simulink model "simscape_final"  (R2023a)
settings: Solver=ode23tb  StartTime=0.0  StopTime=0.15  RelTol=1e-3
PreLoadFcn:
  | clear;
  | clc;
  | %load('70PVArrayExperimentalData.mat');
  | 
  | MPPT_IncCond=Simulink.Variant('MPPT_MODE==1')
  | MPPT_PandO=Simulink.Variant('MPPT_MODE==2')
  | 
  | MPPT_MODE=2
  | 
  | 
  | Constant_800=Simulink.Variant('Irradiance_Mode==1')
  | Constant_1000=Simulink.Variant('Irradiance_Mode==2')
  | Step=Simulink.Variant('Irradiance_Mode==3')
  | Step2=Simulink.Variant('Irradiance_Mode==4')
  | Irradiance_Mode=4
values from neighbouring files (symbols this model uses):
  ArrayCurrent2 = [3.444 3.44193327944 3.44169340802 3.44145256796 3.44121172825 3.44097088836 3.44073004827 3.44048920799 3.4402483675 3.44000752679 3.43976668584 3.43952584466 ... (5005 elements, 385x13)]    [InitPVArrayData.mat]
  ArrayVoltage = [0 0.1 0.2 0.3 0.4 0.5 0.6 0.7 0.8 0.9 1 1.1 ... (215 elements, 1x215)]    [25PVArrayExperimentalData.mat]    (also in 70PVArrayExperimentalData.mat = [0 0.1 0.2 0.3 0.4 0.5 0.6 0.7 0.8 0.9 1 1.1 ... (183 elemen; InitPVArrayData.mat = [0 0.1 0.2 0.3 0.4 0.5 0.6 0.7 0.8 0.9 1 1.1 ... (385 elemen)
  Irradiance = [400 450 500 550 600 650 700 750 800 850 900 950 ... (17 elements, 1x17)]    [25PVArrayExperimentalData.mat]    (also in 70PVArrayExperimentalData.mat; InitPVArrayData.mat = [400 450 500 550 600 650 700 750 800 850 900 950 ... (13 ele)
undefined symbols (not defined in the file or in its folder): sigbuilder_block
libraries: spsSeriesRLCBranchLib x6, SignalEditorBlockLib x4, spsVoltageMeasurementLib x4, simulink x3, spsDiodeLib x3, spsMosfetLib x3, spsCurrentMeasurementLib x2, spsControlledCurrentSourceLib x2, spspowerguiLib x1
settings Model: SimulationMode=accelerator  Creator=gabrielcrisan  LastModifiedBy=gabrielcrisan

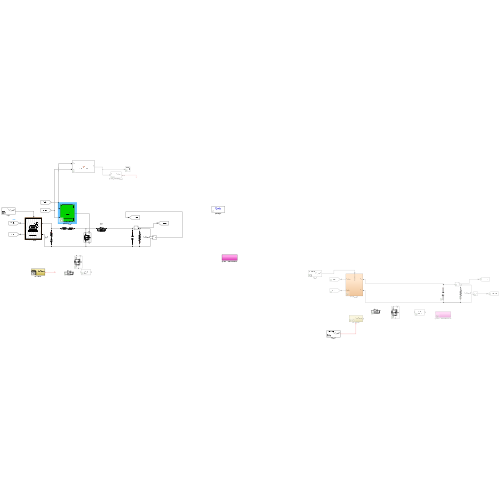
[thumbnail: Simulink's stored preview of the top-level diagram]
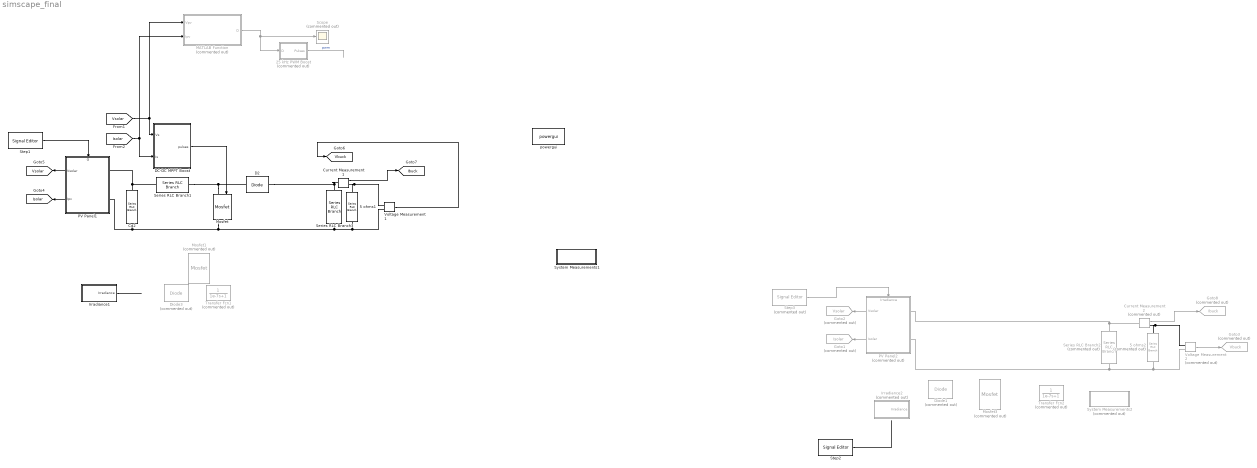
== system simscape_final ==
  25 kHz PWM Boost : Subsystem  Commented=on  mask{Freq=25000}
      mask prompts: Freq "Frequency (Hz)"
  5 ohms1 : spsSeriesRLCBranchLib/Series RLC Branch  LConnTagsString=__new0  RConnTagsString=__new0  BranchType=R  Resistance=15  Inductance=0  SetiL0=off  InitialCurrent=0  Capacitance=100e-6  Setx0=off  InitialVoltage=0  Measurements=Branch voltage and current
  5 ohms2 : spsSeriesRLCBranchLib/Series RLC Branch  Commented=on  LConnTagsString=__new0  RConnTagsString=__new0  BranchType=R  Resistance=15  Inductance=0  SetiL0=off  InitialCurrent=0  Capacitance=100e-6  Setx0=off  InitialVoltage=0  Measurements=Branch voltage and current
  Cg2 : spsSeriesRLCBranchLib/Series RLC Branch  LConnTagsString=__new0  RConnTagsString=__new0  BranchType=RC  Resistance=0.000001  Inductance=0  SetiL0=off  InitialCurrent=0  Capacitance=100e-6  Setx0=off  InitialVoltage=0  Measurements=None
  Current Measurement1 : spsCurrentMeasurementLib/Current Measurement  PhasorSimulation=off  OutputType=Complex  PSBequivalent=0
  Current Measurement2 : spsCurrentMeasurementLib/Current Measurement  Commented=on  PhasorSimulation=off  OutputType=Complex  PSBequivalent=0
  D2 : spsDiodeLib/Diode  Ron=0.001  Lon=0  Vf=0.8  IC=0  UseSnubber=off  Rs=500  Cs=250e-9  Measurements=off
  DC-DC MPPT Boost : Subsystem  Variant=on
      mask Display: image('$imagefile'); % Use "Edit Image" on toolstrip to change.
  Diode1 : spsDiodeLib/Diode  Commented=on  Ron=0.001  Lon=0  Vf=0.8  IC=0  UseSnubber=0  Rs=500  Cs=250e-9  Measurements=off
  Diode3 : spsDiodeLib/Diode  Commented=on  Ron=0.001  Lon=0  Vf=0.8  IC=0  UseSnubber=0  Rs=500  Cs=250e-9  Measurements=off
  Goto1 : Goto  Commented=on  GotoTag=Isolar  TagVisibility=global
  Goto2 : Goto  Commented=on  GotoTag=Vsolar  TagVisibility=global
  Goto3 : Goto  Commented=on  GotoTag=Vbuck  TagVisibility=global
  Goto8 : Goto  Commented=on  GotoTag=Ibuck  TagVisibility=global
  Irradiance1 : Subsystem  Variant=on
  Irradiance2 : Subsystem  Commented=on  Variant=on
  MATLAB Function : MATLAB Function  Commented=on  TreatAsAtomicUnit=on
  Mosfet : spsMosfetLib/Mosfet  Ron=0.001  Lon=0  Rd=0.001  Vfd=0  IC=0  Rs=1e5  Cs=inf  Measurements=on
  Mosfet1 : spsMosfetLib/Mosfet  Commented=on  Ron=0.1  Lon=0  Rd=0.01  Vfd=0  IC=0  Rs=1e5  Cs=inf  Measurements=off
  Mosfet3 : spsMosfetLib/Mosfet  Commented=on  Ron=0.1  Lon=0  Rd=0.01  Vfd=0  IC=0  Rs=1e5  Cs=inf  Measurements=off
  PV Panel1 : Subsystem
      settings: PortSchema="{\"entries\":[{\"content\":{\"sides\":[{\"content\":{\"connectorIds\":[\"LConn1\",\"LConn2\"]},\"type\":\"ConnectorPlacement.EquallySpacedRectSide\",\"uuid\":\"43992eb9-8484-404f-bfb9-e76ffbcbe789\"},{\"content\":{\"connectorIds\":[\"Out1\",\"Out2\"],\"side\":\"RIGHT\"},\"type\":\"ConnectorPlacement.EquallySpacedRectSide\",\"uuid\":\"a1e110c3-733a-48a0-9f21-72c7769fefeb\"},{\"content\":{\"connectorIds\":[\"In1\"],\"side\":\"TOP\"},\"type\":\"ConnectorPlacement.EquallySpacedRectSide\",\"uuid\":\"462cd67a-8eaa-46f4-b7ed-de8fc592bb6c\"}]},\"type\":\"ConnectorPlacement.EquallySpacedConnector\",\"uuid\":\"36390758-a197-45c1-a178-dbe841a9808e\"}],\"packageUris\":[\"http://schema.mathworks.com/mf0/Connector/R2020b\"],\"version\":\"1.0\"}"
      mask Display: image('$imagefile'); % Use "Edit Image" on toolstrip to change.
  PV Panel2 : Subsystem  Commented=on
      settings: PortSchema="{\"entries\":[{\"content\":{\"sides\":[{\"content\":{\"connectorIds\":[\"LConn1\",\"LConn2\"]},\"type\":\"ConnectorPlacement.EquallySpacedRectSide\",\"uuid\":\"d9bf1892-3ed2-4c2d-93df-cd3e3a16e4c3\"},{\"content\":{\"connectorIds\":[\"Out1\",\"Out2\"],\"side\":\"RIGHT\"},\"type\":\"ConnectorPlacement.EquallySpacedRectSide\",\"uuid\":\"0c4558bb-5c04-452d-a739-3e65dffd873d\"},{\"content\":{\"connectorIds\":[\"In1\"],\"side\":\"TOP\"},\"type\":\"ConnectorPlacement.EquallySpacedRectSide\",\"uuid\":\"688d7f81-1212-47ef-a811-baa40651be20\"}]},\"type\":\"ConnectorPlacement.EquallySpacedConnector\",\"uuid\":\"9406dafc-96f7-4a37-8af1-81987149706d\"}],\"packageUris\":[\"http://schema.mathworks.com/mf0/Connector/R2020b\"],\"version\":\"1.0\"}"
  Scope : Scope  Commented=on
  Series RLC Branch1 : spsSeriesRLCBranchLib/Series RLC Branch  LConnTagsString=__new0  RConnTagsString=__new0  BranchType=RL  Resistance=0.001  Inductance=200e-6  SetiL0=off  InitialCurrent=0  Capacitance=100e-6  Setx0=off  InitialVoltage=0  Measurements=None
  Series RLC Branch2 : spsSeriesRLCBranchLib/Series RLC Branch  Commented=on  LConnTagsString=__new0  RConnTagsString=__new0  BranchType=C  Resistance=1e-6  Inductance=0  SetiL0=off  InitialCurrent=0  Capacitance=50e-6  Setx0=off  InitialVoltage=0  Measurements=None
  Series RLC Branch3 : spsSeriesRLCBranchLib/Series RLC Branch  LConnTagsString=__new0  RConnTagsString=__new0  BranchType=C  Resistance=1e-6  Inductance=0  SetiL0=off  InitialCurrent=0  Capacitance=50e-6  Setx0=off  InitialVoltage=0  Measurements=None
  Step1 : SignalEditorBlockLib/Signal Editor  VariantControl=Choice  FileName=IR_scenario.mat  ActiveScenario=Scenario  ActiveSignal=Ir1_rand  IsBus=off  OutputBusObjectStr=Bus: BusObject  SampleTime=0  Interpolate=off  ZeroCross=off  OutputAfterFinalValue=Setting to zero  Unit=inherit  PreserveSignalName=on  ApplySigPropsToAllScenarios=on
  Step2 : SignalEditorBlockLib/Signal Editor  VariantControl=Choice  FileName=IR_scenario.mat  ActiveScenario=Scenario  ActiveSignal=Ir1_rand  IsBus=off  OutputBusObjectStr=Bus: BusObject  SampleTime=0  Interpolate=off  ZeroCross=off  OutputAfterFinalValue=Setting to zero  Unit=inherit  PreserveSignalName=on  ApplySigPropsToAllScenarios=on
  Step3 : SignalEditorBlockLib/Signal Editor  Commented=on  VariantControl=Choice  FileName=IR_scenario.mat  ActiveScenario=Scenario  ActiveSignal=Ir1_rand  IsBus=off  OutputBusObjectStr=Bus: BusObject  SampleTime=0  Interpolate=off  ZeroCross=off  OutputAfterFinalValue=Setting to zero  Unit=inherit  PreserveSignalName=on  ApplySigPropsToAllScenarios=on
  System Measurements1 : Subsystem
  System Measurements2 : Subsystem  Commented=on
  Transfer Fcn1 : TransferFcn  Commented=on  Denominator=[1e-7 1]
  Transfer Fcn2 : TransferFcn  Commented=on  Denominator=[1e-7 1]
  Voltage Measurement1 : spsVoltageMeasurementLib/Voltage Measurement  PhasorSimulation=off  OutputType=Complex  PSBequivalent=0
  Voltage Measurement2 : spsVoltageMeasurementLib/Voltage Measurement  Commented=on  PhasorSimulation=off  OutputType=Complex  PSBequivalent=0
  powergui : spspowerguiLib/powergui  Priority=1  SimulationMode=Discrete  SampleTime=1e-7  frequency=60  Iterations=50  frequencyindice=0  Pbase=100e6  ErrMax=1e-4  UnitsV=kV  UnitsW=MW  buscounter=0  FunctionMessages=off  echomessages=off  EnableUseOfTLC=off  CurrentSourceSwitches=off  DisableSnubberDevices=off  DisableRonSwitches=off  DisableVfSwitches=off  DisplayEquations=off  AutomaticDiscreteSolvers=off  SolverType=Tustin/Backward Euler (TBE)  Interpol=off  ExternalGateDelay=off  methode=off  Ts=100  x0status=blocks  SPID=on  SwTol=0  HookPort=off  NonlinearTolerance=1e-4  nMaxIteration=100  ContinueOnMaxIteration=off  RestoreLinks=warning  ResistiveCurrentMeasurement=off  Frange=[0:2:500]  Ylog=off  Xlog=on  ShowGrid=off  save=off  variable=ZData  structure=0  ZoomFFT=off  StartTime=0.0  cycles=1  DisplayStyle=1  fundamental=60  FreqAxis=off  MaxFrequency=1000  frequencyindicesteady=1  RmsSteady=1  display=off
  tag scope: Ibuck=global, Isolar=global, Vbuck=global, Vsolar=global
  wires:
  [Vsolar] -> MATLAB Function/1(Vpv), DC-DC MPPT Boost/1(Vs)
  PV Panel1/1(Vsolar) -> [Vsolar]
  Irradiance1/1(Irradiance) -> ?
  MATLAB Function/1(D) -> Scope/1, 25 kHz PWM Boost/1(D)
  [Isolar] -> MATLAB Function/2(Ipv), DC-DC MPPT Boost/2(Is)
  Voltage Measurement1/1 -> [Vbuck]
  Current Measurement1/1 -> [Ibuck]
  PV Panel1/2(Ipv) -> [Isolar]
  25 kHz PWM Boost/1(Pulses) -> ?  "pwm"
  DC-DC MPPT Boost/1(pulses) -> Mosfet/1
  PV Panel2/1(Vsolar) -> Goto2/1
  PV Panel2/2(Isolar) -> Goto1/1
  Voltage Measurement2/1 -> Goto3/1
  Current Measurement2/1 -> Goto8/1
  Step2/1 -> ?
  Step1/1 -> PV Panel1/1(G)
  Step3/1 -> PV Panel2/1(Irradiance)
  connections:
  PV Panel1/LConn2 -- Cg2/RConn1 -- Mosfet/RConn1 -- 5 ohms1/LConn1 -- Voltage Measurement1/LConn2 -- Series RLC Branch3/RConn1
  PV Panel1/LConn1 -- Series RLC Branch1/RConn1 -- Cg2/LConn1
  D2/RConn1 -- Series RLC Branch3/LConn1 -- Current Measurement1/LConn1
  Mosfet/LConn1 -- Series RLC Branch1/LConn1 -- D2/LConn1
  Voltage Measurement1/LConn1 -- 5 ohms1/RConn1 -- Current Measurement1/RConn1
  Current Measurement2/LConn1 -- PV Panel2/LConn1 -- Series RLC Branch2/LConn1
  Voltage Measurement2/LConn1 -- 5 ohms2/RConn1 -- Current Measurement2/RConn1
  Voltage Measurement2/LConn2 -- 5 ohms2/LConn1 -- Series RLC Branch2/RConn1 -- PV Panel2/LConn2

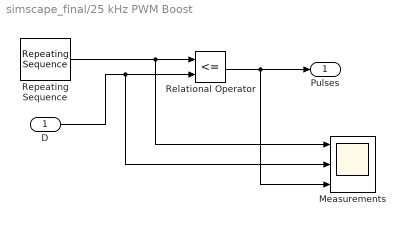
== system simscape_final/25 kHz PWM Boost ==
  D : Inport
  Measurements : Scope  NumInputPorts=3
  Relational Operator : RelationalOperator  Operator=<=  OutDataTypeStr=boolean  ZeroCross=off  InputSameDT=off
  Repeating Sequence : simulink/Sources/Repeating Sequence  rep_seq_t="[0  1/Freq]"  rep_seq_y=[0 1]
  Pulses : Outport
  wires:
  Repeating Sequence/1 -> Measurements/1, Relational Operator/1
  Relational Operator/1 -> Measurements/3, Pulses/1
  D/1 -> Measurements/2, Relational Operator/2

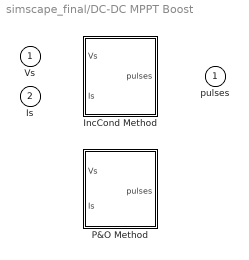
== system simscape_final/DC-DC MPPT Boost ==
  Vs : Inport
  Is : Inport  Port=2
  IncCond Method : Subsystem  VariantControl=MPPT_IncCond
  P&O Method : Subsystem  VariantControl=MPPT_PandO
  pulses : Outport

== system simscape_final/Irradiance1 ==
  Constant 1000 : Subsystem  Tag=STV Subsys  LoadFcn=sigbuilder_block('load');  StartFcn=sigbuilder_block('start');  StopFcn=sigbuilder_block('stop');  ClipboardFcn=sigbuilder_block('clipboard');  VariantControl=Constant_1000  mask(Sigbuilder block){tuvar=[0:10]}
      mask help: Simulink:masks:SigbuilderBlock_MD
      mask init:
      | if ~strcmp(get_param(bdroot(gcbh),'SimulationStatus'),'stopped') tuvar = sigbuilder_block('maskInit'); end
      settings: CopyFcn=sigbuilder_block('copy');  DeleteFcn=sigbuilder_block('delete');  ModelCloseFcn=sigbuilder_block('modelClose');  PreSaveFcn=sigbuilder_block('preSave');  PauseFcn=sigbuilder_block('pause')  ContinueFcn=sigbuilder_block('continue')  NameChangeFcn=sigbuilder_block('namechange');  OpenFcn=sigbuilder_block('open',[365.25 126 411.75 327.75 ]);  CloseFcn=sigbuilder_block('close');
      mask Display: plot(0, 0, 100, 100,[2, 2, 32, 32, 2], [68, 8, 8, 68, 68],[32, 2], [38, 38], [32, 19, 2],[53, 60, 44], [32, 17, 17, 2],[16, 16, 31, 31]);txt = getActiveGroup(gcbh);text(2, 100, txt,'verticalAlignment', 'top');
  "Constant 800 " : Subsystem  Tag=STV Subsys  LoadFcn=sigbuilder_block('load');  StartFcn=sigbuilder_block('start');  StopFcn=sigbuilder_block('stop');  ClipboardFcn=sigbuilder_block('clipboard');  VariantControl=Constant_800  mask(Sigbuilder block){tuvar=[0:10]}
      mask help: Simulink:masks:SigbuilderBlock_MD
      mask init:
      | if ~strcmp(get_param(bdroot(gcbh),'SimulationStatus'),'stopped') tuvar = sigbuilder_block('maskInit'); end
      settings: CopyFcn=sigbuilder_block('copy');  DeleteFcn=sigbuilder_block('delete');  ModelCloseFcn=sigbuilder_block('modelClose');  PreSaveFcn=sigbuilder_block('preSave');  PauseFcn=sigbuilder_block('pause')  ContinueFcn=sigbuilder_block('continue')  NameChangeFcn=sigbuilder_block('namechange');  OpenFcn=sigbuilder_block('open',[365.25 126 411.75 327.75 ]);  CloseFcn=sigbuilder_block('close');
      mask Display: plot(0, 0, 100, 100,[2, 2, 32, 32, 2], [68, 8, 8, 68, 68],[32, 2], [38, 38], [32, 19, 2],[53, 60, 44], [32, 17, 17, 2],[16, 16, 31, 31]);txt = getActiveGroup(gcbh);text(2, 100, txt,'verticalAlignment', 'top');
  Step : Subsystem  Tag=STV Subsys  LoadFcn=sigbuilder_block('load');  StartFcn=sigbuilder_block('start');  StopFcn=sigbuilder_block('stop');  ClipboardFcn=sigbuilder_block('clipboard');  VariantControl=Step  mask(Sigbuilder block){tuvar=[0:10]}
      mask help: Simulink:masks:SigbuilderBlock_MD
      mask init:
      | if ~strcmp(get_param(bdroot(gcbh),'SimulationStatus'),'stopped') tuvar = sigbuilder_block('maskInit'); end
      settings: CopyFcn=sigbuilder_block('copy');  DeleteFcn=sigbuilder_block('delete');  ModelCloseFcn=sigbuilder_block('modelClose');  PreSaveFcn=sigbuilder_block('preSave');  PauseFcn=sigbuilder_block('pause')  ContinueFcn=sigbuilder_block('continue')  NameChangeFcn=sigbuilder_block('namechange');  OpenFcn=sigbuilder_block('open',[135.75 161.25 411.75 327.75 ]);  CloseFcn=sigbuilder_block('close');
      mask Display: plot(0, 0, 100, 100,[2, 2, 32, 32, 2], [68, 8, 8, 68, 68],[32, 2], [38, 38], [32, 19, 2],[53, 60, 44], [32, 17, 17, 2],[16, 16, 31, 31]);txt = getActiveGroup(gcbh);text(2, 100, txt,'verticalAlignment', 'top');
  Irradiance : Outport

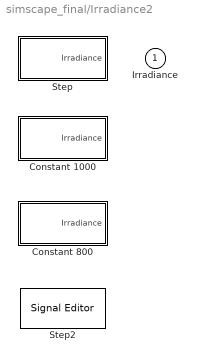
== system simscape_final/Irradiance2 ==
  Constant 1000 : Subsystem  Tag=STV Subsys  LoadFcn=sigbuilder_block('load');  StartFcn=sigbuilder_block('start');  StopFcn=sigbuilder_block('stop');  ClipboardFcn=sigbuilder_block('clipboard');  VariantControl=Constant_1000  mask(Sigbuilder block){tuvar=[0:10]}
      mask help: Simulink:masks:SigbuilderBlock_MD
      mask init:
      | if ~strcmp(get_param(bdroot(gcbh),'SimulationStatus'),'stopped') tuvar = sigbuilder_block('maskInit'); end
      settings: CopyFcn=sigbuilder_block('copy');  DeleteFcn=sigbuilder_block('delete');  ModelCloseFcn=sigbuilder_block('modelClose');  PreSaveFcn=sigbuilder_block('preSave');  PauseFcn=sigbuilder_block('pause')  ContinueFcn=sigbuilder_block('continue')  NameChangeFcn=sigbuilder_block('namechange');  OpenFcn=sigbuilder_block('open',[365.25 126 411.75 327.75 ]);  CloseFcn=sigbuilder_block('close');
      mask Display: plot(0, 0, 100, 100,[2, 2, 32, 32, 2], [68, 8, 8, 68, 68],[32, 2], [38, 38], [32, 19, 2],[53, 60, 44], [32, 17, 17, 2],[16, 16, 31, 31]);txt = getActiveGroup(gcbh);text(2, 100, txt,'verticalAlignment', 'top');
  "Constant 800 " : Subsystem  Tag=STV Subsys  LoadFcn=sigbuilder_block('load');  StartFcn=sigbuilder_block('start');  StopFcn=sigbuilder_block('stop');  ClipboardFcn=sigbuilder_block('clipboard');  VariantControl=Constant_800  mask(Sigbuilder block){tuvar=[0:10]}
      mask help: Simulink:masks:SigbuilderBlock_MD
      mask init:
      | if ~strcmp(get_param(bdroot(gcbh),'SimulationStatus'),'stopped') tuvar = sigbuilder_block('maskInit'); end
      settings: CopyFcn=sigbuilder_block('copy');  DeleteFcn=sigbuilder_block('delete');  ModelCloseFcn=sigbuilder_block('modelClose');  PreSaveFcn=sigbuilder_block('preSave');  PauseFcn=sigbuilder_block('pause')  ContinueFcn=sigbuilder_block('continue')  NameChangeFcn=sigbuilder_block('namechange');  OpenFcn=sigbuilder_block('open',[365.25 126 411.75 327.75 ]);  CloseFcn=sigbuilder_block('close');
      mask Display: plot(0, 0, 100, 100,[2, 2, 32, 32, 2], [68, 8, 8, 68, 68],[32, 2], [38, 38], [32, 19, 2],[53, 60, 44], [32, 17, 17, 2],[16, 16, 31, 31]);txt = getActiveGroup(gcbh);text(2, 100, txt,'verticalAlignment', 'top');
  Step : Subsystem  Tag=STV Subsys  LoadFcn=sigbuilder_block('load');  StartFcn=sigbuilder_block('start');  StopFcn=sigbuilder_block('stop');  ClipboardFcn=sigbuilder_block('clipboard');  VariantControl=Step  mask(Sigbuilder block){tuvar=[0:10]}
      mask help: Simulink:masks:SigbuilderBlock_MD
      mask init:
      | if ~strcmp(get_param(bdroot(gcbh),'SimulationStatus'),'stopped') tuvar = sigbuilder_block('maskInit'); end
      settings: CopyFcn=sigbuilder_block('copy');  DeleteFcn=sigbuilder_block('delete');  ModelCloseFcn=sigbuilder_block('modelClose');  PreSaveFcn=sigbuilder_block('preSave');  PauseFcn=sigbuilder_block('pause')  ContinueFcn=sigbuilder_block('continue')  NameChangeFcn=sigbuilder_block('namechange');  OpenFcn=sigbuilder_block('open',[135.75 161.25 411.75 327.75 ]);  CloseFcn=sigbuilder_block('close');
      mask Display: plot(0, 0, 100, 100,[2, 2, 32, 32, 2], [68, 8, 8, 68, 68],[32, 2], [38, 38], [32, 19, 2],[53, 60, 44], [32, 17, 17, 2],[16, 16, 31, 31]);txt = getActiveGroup(gcbh);text(2, 100, txt,'verticalAlignment', 'top');
  Step2 : SignalEditorBlockLib/Signal Editor  VariantControl=Choice  FileName=IR_scenario.mat  ActiveScenario=Scenario  ActiveSignal=Ir1_rand  IsBus=off  OutputBusObjectStr=Bus: BusObject  SampleTime=0  Interpolate=off  ZeroCross=off  OutputAfterFinalValue=Setting to zero  Unit=inherit  PreserveSignalName=on  ApplySigPropsToAllScenarios=on
  Irradiance : Outport

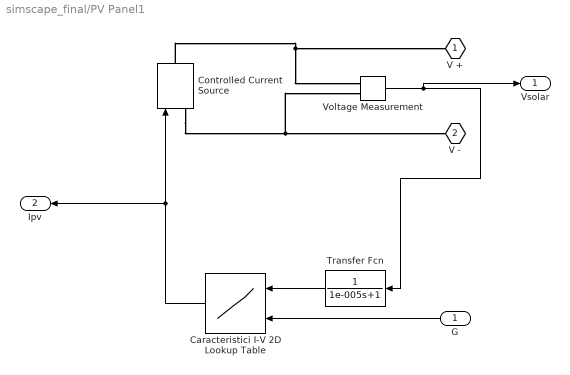
== system simscape_final/PV Panel1 ==
  G : Inport
  Caracteristici I-V 2D Lookup Table : Lookup_n-D  BreakpointsForDimension1=ArrayVoltage  BreakpointsForDimension2=Irradiance  Table=ArrayCurrent2  RndMeth=Simplest
      settings: InputPortMap=u0,u1
      mask Display: image('$imagefile'); % Use "Edit Image" on toolstrip to change.
  Controlled Current Source : spsControlledCurrentSourceLib/Controlled Current Source  Initialize=on  Source_Type=DC  Amplitude=0  Phase=0  Frequency=0  Measurements=None
  Transfer Fcn : TransferFcn  Denominator=[1e-005 1]
      mask Display: image('$imagefile'); % Use "Edit Image" on toolstrip to change.
  Voltage Measurement : spsVoltageMeasurementLib/Voltage Measurement  PhasorSimulation=off  OutputType=Complex  PSBequivalent=0
  V + : PMIOPort  Side=Left
  V - : PMIOPort  Port=2  Side=Left
  Vsolar : Outport
  Ipv : Outport  Port=2
  wires:
  G/1 -> Caracteristici I-V 2D Lookup Table/2
  Voltage Measurement/1 -> Transfer Fcn/1, Vsolar/1
  Transfer Fcn/1 -> Caracteristici I-V 2D Lookup Table/1
  Caracteristici I-V 2D Lookup Table/1 -> Ipv/1, Controlled Current Source/1
  connections:
  Controlled Current Source/LConn1 -- V -/RConn1 -- Voltage Measurement/LConn2
  Controlled Current Source/RConn1 -- V +/RConn1 -- Voltage Measurement/LConn1

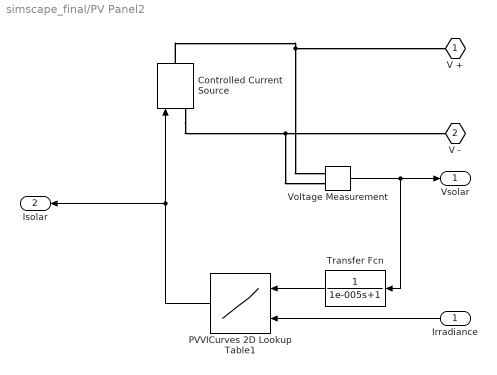
== system simscape_final/PV Panel2 ==
  Irradiance : Inport
  Controlled Current Source : spsControlledCurrentSourceLib/Controlled Current Source  Initialize=on  Source_Type=DC  Amplitude=0  Phase=0  Frequency=0  Measurements=None
  PVVICurves 2D Lookup Table1 : Lookup_n-D  BreakpointsForDimension1=ArrayVoltage  BreakpointsForDimension2=Irradiance  Table=ArrayCurrent2  RndMeth=Simplest
      settings: InputPortMap=u0,u1
  Transfer Fcn : TransferFcn  Denominator=[1e-005 1]
  Voltage Measurement : spsVoltageMeasurementLib/Voltage Measurement  PhasorSimulation=off  OutputType=Complex  PSBequivalent=0
  V + : PMIOPort  Side=Left
  V - : PMIOPort  Port=2  Side=Left
  Vsolar : Outport
  Isolar : Outport  Port=2
  wires:
  Irradiance/1 -> PVVICurves 2D Lookup Table1/2
  Voltage Measurement/1 -> Vsolar/1, Transfer Fcn/1
  Transfer Fcn/1 -> PVVICurves 2D Lookup Table1/1
  PVVICurves 2D Lookup Table1/1 -> Isolar/1, Controlled Current Source/1
  connections:
  Controlled Current Source/LConn1 -- V -/RConn1 -- Voltage Measurement/LConn2
  Controlled Current Source/RConn1 -- V +/RConn1 -- Voltage Measurement/LConn1

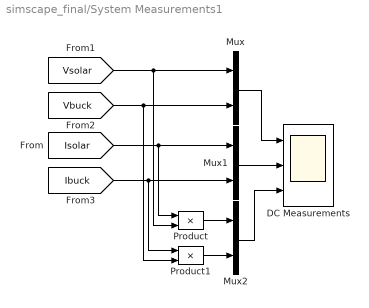
== system simscape_final/System Measurements1 ==
  DC Measurements : Scope  NumInputPorts=3
  Mux : Mux  Inputs=2
  Mux1 : Mux  Inputs=2
  Mux2 : Mux  Inputs=2
  Product : Product  RndMeth=Zero
  Product1 : Product  RndMeth=Zero
  wires:
  Mux/1 -> DC Measurements/1
  [Isolar] -> Mux1/1, Product/1
  Product/1 -> Mux2/1
  Mux1/1 -> DC Measurements/2
  Product1/1 -> Mux2/2
  [Vbuck] -> Mux/2, Product1/2
  Mux2/1 -> DC Measurements/3
  [Vsolar] -> Mux/1, Product/2
  [Ibuck] -> Mux1/2, Product1/1

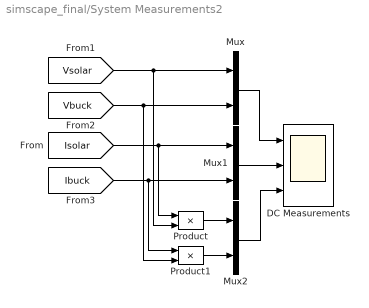
== system simscape_final/System Measurements2 ==
  DC Measurements : Scope  NumInputPorts=3
  Mux : Mux  Inputs=2
  Mux1 : Mux  Inputs=2
  Mux2 : Mux  Inputs=2
  Product : Product  RndMeth=Zero
  Product1 : Product  RndMeth=Zero
  wires:
  Mux/1 -> DC Measurements/1
  [Isolar] -> Mux1/1, Product/1
  Product/1 -> Mux2/1
  Mux1/1 -> DC Measurements/2
  Product1/1 -> Mux2/2
  [Vbuck] -> Mux/2, Product1/2
  Mux2/1 -> DC Measurements/3
  [Vsolar] -> Mux/1, Product/2
  [Ibuck] -> Mux1/2, Product1/1

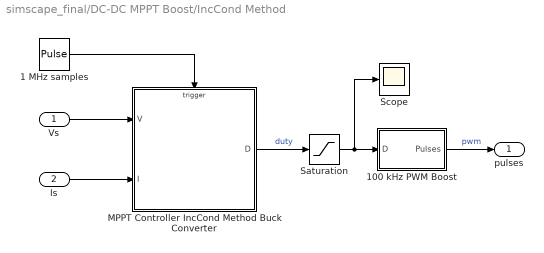
== system simscape_final/DC-DC MPPT Boost/IncCond Method ==
  Vs : Inport
  Is : Inport  Port=2
  1 MHz samples : DiscretePulseGenerator  PulseType=Time based  Period=0.000001  PulseWidth=5
  100 kHz PWM Boost : Subsystem  mask{Freq=100000}
      mask prompts: Freq "Frequency (Hz)"
  MPPT Controller IncCond Method Buck Converter : Stateflow chart  TreatAsAtomicUnit=on
  Saturation : Saturate  UpperLimit=1  LowerLimit=0  OutMin=[0]  OutMax=[1]
  Scope : Scope
  pulses : Outport
  wires:
  Vs/1 -> MPPT Controller IncCond Method Buck Converter/1(V)
  MPPT Controller IncCond Method Buck Converter/1(D) -> Saturation/1  "duty"
  100 kHz PWM Boost/1(Pulses) -> pulses/1  "pwm"
  1 MHz samples/1 -> MPPT Controller IncCond Method Buck Converter/Trigger
  Saturation/1 -> Scope/1, 100 kHz PWM Boost/1(D)
  Is/1 -> MPPT Controller IncCond Method Buck Converter/2(I)

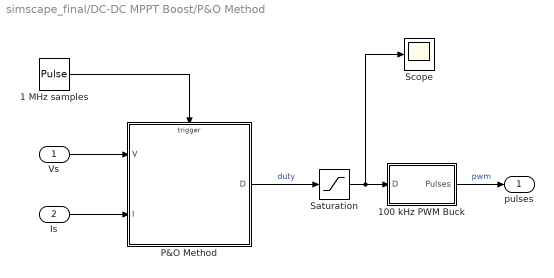
== system simscape_final/DC-DC MPPT Boost/P&O Method ==
  Vs : Inport
  Is : Inport  Port=2
  1 MHz samples : DiscretePulseGenerator  PulseType=Time based  Period=0.000001  PulseWidth=5
  100 kHz PWM Buck : Subsystem  mask{Freq=10000}
      mask prompts: Freq "Frequency (Hz)"
  P&O Method : Stateflow chart  TreatAsAtomicUnit=on
  Saturation : Saturate  UpperLimit=1  LowerLimit=0  OutMin=[0]  OutMax=[1]
  Scope : Scope
  pulses : Outport
  wires:
  100 kHz PWM Buck/1(Pulses) -> pulses/1  "pwm"
  Is/1 -> P&O Method/2(I)
  Vs/1 -> P&O Method/1(V)
  Saturation/1 -> Scope/1, 100 kHz PWM Buck/1(D)
  1 MHz samples/1 -> P&O Method/Trigger
  P&O Method/1(D) -> Saturation/1  "duty"

== system simscape_final/Irradiance1/Constant 1000 ==
  Demux : Demux  Tag=STV Demux  Outputs=1
      settings: DisplayOption=none
  FromWs : FromWorkspace  Tag=STV FromWs  VariableName=tuvar
      SigBuilderData=|
      | common.afterFinalStr = 'Extrapolate'
      | common.sampleTime = 0
      | dataSet.timeRange = [0 0.1]
      | dataSet.name = '1000'
      | sbobj.Groups.Name = '1000'
      | sbobj.Groups.Signals.Name = 'Irradiance'
      | sbobj.Groups.Signals.XData = [0 0.1]
      | sbobj.Groups.Signals.YData = [1000 1000]
      | sbobj.Groups.TimeRange = [0 0.1]
  Irradiance : Outport  Tag=STV Outport
  wires:
  Demux/1 -> Irradiance/1
  FromWs/1 -> Demux/1

== system simscape_final/Irradiance1/Constant 800  ==
  Demux : Demux  Tag=STV Demux  Outputs=1
      settings: DisplayOption=none
  FromWs : FromWorkspace  Tag=STV FromWs  VariableName=tuvar
      SigBuilderData=|
      | common.afterFinalStr = 'Extrapolate'
      | common.sampleTime = 0
      | dataSet.timeRange = [0 0.1]
      | dataSet.name = '800'
      | sbobj.Groups.Name = '800'
      | sbobj.Groups.Signals.Name = 'Irradiance'
      | sbobj.Groups.Signals.XData = [0 0.1]
      | sbobj.Groups.Signals.YData = [800 800]
      | sbobj.Groups.TimeRange = [0 0.1]
  Irradiance : Outport  Tag=STV Outport
  wires:
  Demux/1 -> Irradiance/1
  FromWs/1 -> Demux/1

== system simscape_final/Irradiance1/Step ==
  Demux : Demux  Tag=STV Demux  Outputs=1
      settings: DisplayOption=none
  FromWs : FromWorkspace  Tag=STV FromWs  VariableName=tuvar
      SigBuilderData=|
      | common.afterFinalStr = 'Extrapolate'
      | common.sampleTime = 0
      | dataSet.timeRange = [0 0.1]
      | dataSet.name = 'Step'
      | sbobj.Groups.Name = 'Step'
      | sbobj.Groups.Signals.Name = 'Irradiance'
      | sbobj.Groups.Signals.XData = [0 0.02 0.02 0.04 0.04 0.06 0.06 0.08 0.08 0.1]
      | sbobj.Groups.Signals.YData = [800 800 600 600 1000 1000 800 800 600 600]
      | sbobj.Groups.TimeRange = [0 0.1]
  Irradiance : Outport  Tag=STV Outport
  wires:
  Demux/1 -> Irradiance/1
  FromWs/1 -> Demux/1

== system simscape_final/Irradiance2/Constant 1000 ==
  Demux : Demux  Tag=STV Demux  Outputs=1
      settings: DisplayOption=none
  FromWs : FromWorkspace  Tag=STV FromWs  VariableName=tuvar
      SigBuilderData=|
      | common.afterFinalStr = 'Extrapolate'
      | common.sampleTime = 0
      | dataSet.timeRange = [0 0.1]
      | dataSet.name = '1000'
      | sbobj.Groups.Name = '1000'
      | sbobj.Groups.Signals.Name = 'Irradiance'
      | sbobj.Groups.Signals.XData = [0 0.1]
      | sbobj.Groups.Signals.YData = [1000 1000]
      | sbobj.Groups.TimeRange = [0 0.1]
  Irradiance : Outport  Tag=STV Outport
  wires:
  Demux/1 -> Irradiance/1
  FromWs/1 -> Demux/1

== system simscape_final/Irradiance2/Constant 800  ==
  Demux : Demux  Tag=STV Demux  Outputs=1
      settings: DisplayOption=none
  FromWs : FromWorkspace  Tag=STV FromWs  VariableName=tuvar
      SigBuilderData=|
      | common.afterFinalStr = 'Extrapolate'
      | common.sampleTime = 0
      | dataSet.timeRange = [0 0.1]
      | dataSet.name = '800'
      | sbobj.Groups.Name = '800'
      | sbobj.Groups.Signals.Name = 'Irradiance'
      | sbobj.Groups.Signals.XData = [0 0.1]
      | sbobj.Groups.Signals.YData = [800 800]
      | sbobj.Groups.TimeRange = [0 0.1]
  Irradiance : Outport  Tag=STV Outport
  wires:
  Demux/1 -> Irradiance/1
  FromWs/1 -> Demux/1

== system simscape_final/Irradiance2/Step ==
  Demux : Demux  Tag=STV Demux  Outputs=1
      settings: DisplayOption=none
  FromWs : FromWorkspace  Tag=STV FromWs  VariableName=tuvar
      SigBuilderData=|
      | common.afterFinalStr = 'Extrapolate'
      | common.sampleTime = 0
      | dataSet.timeRange = [0 0.1]
      | dataSet.name = 'Step'
      | sbobj.Groups.Name = 'Step'
      | sbobj.Groups.Signals.Name = 'Irradiance'
      | sbobj.Groups.Signals.XData = [0 0.02 0.02 0.04 0.04 0.06 0.06 0.08 0.08 0.1]
      | sbobj.Groups.Signals.YData = [800 800 600 600 1000 1000 800 800 600 600]
      | sbobj.Groups.TimeRange = [0 0.1]
  Irradiance : Outport  Tag=STV Outport
  wires:
  Demux/1 -> Irradiance/1
  FromWs/1 -> Demux/1

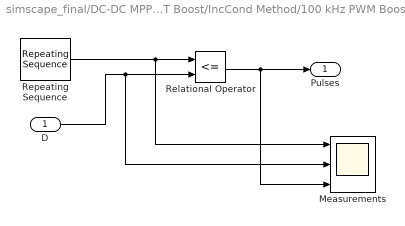
== system simscape_final/DC-DC MPPT Boost/IncCond Method/100 kHz PWM Boost ==
  D : Inport
  Measurements : Scope  NumInputPorts=3
  Relational Operator : RelationalOperator  Operator=<=  OutDataTypeStr=boolean  ZeroCross=off  InputSameDT=off
  Repeating Sequence : simulink/Sources/Repeating Sequence  rep_seq_t="[0  1/Freq]"  rep_seq_y=[0 1]
  Pulses : Outport
  wires:
  D/1 -> Relational Operator/2, Measurements/2
  Relational Operator/1 -> Pulses/1, Measurements/3
  Repeating Sequence/1 -> Relational Operator/1, Measurements/1

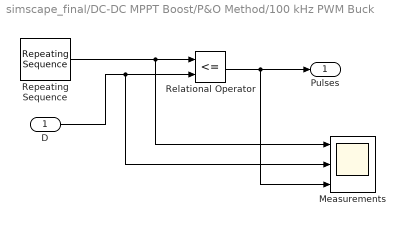
== system simscape_final/DC-DC MPPT Boost/P&O Method/100 kHz PWM Buck ==
  D : Inport
  Measurements : Scope  NumInputPorts=3
  Relational Operator : RelationalOperator  Operator=<=  OutDataTypeStr=boolean  ZeroCross=off  InputSameDT=off
  Repeating Sequence : simulink/Sources/Repeating Sequence  rep_seq_t="[0  1/Freq]"  rep_seq_y=[0 1]
  Pulses : Outport
  wires:
  Repeating Sequence/1 -> Measurements/1, Relational Operator/1
  Relational Operator/1 -> Measurements/3, Pulses/1
  D/1 -> Measurements/2, Relational Operator/2

== stateflow chart simscape_final/DC-DC MPPT Boost/IncCond Method/MPPT Controller IncCond Method Buck Converter ==
  state AVERAGE100SAMPLES
    entry:
    Vsum = 0; Isum = 0; k = 0;
    during:
    Vsum = Vsum + V;
    Isum = Isum + I; k++;
    exit:
    Vavg = Vsum/k;
    Iavg = Isum/k;
  state SAMPLEandCALCULATE
    entry:
    deltaV = Vavg - Vprev;
    deltaI = Iavg - Iprev;
    d = D;
  state DECREMENT
    entry:
    d = d - deltad;
  state INCREMENT
    entry:
    d = d + deltad;
  state RETURN
    entry:
    Vprev = Vavg;
    Iprev = Iavg;
    D = d;
  RETURN -> AVERAGE100SAMPLES
  (default) -> AVERAGE100SAMPLES
  AVERAGE100SAMPLES -> SAMPLEandCALCULATE : after(100,clk)
  SAMPLEandCALCULATE -> (junction 16) [order 1] : [deltaV~=0]
  SAMPLEandCALCULATE -> (junction 17) [order 2] : [deltaV==0]
  (junction 17) -> INCREMENT [order 1] : [deltaI < 0]
  (junction 17) -> RETURN [order 3] : [deltaI == 0]
  (junction 16) -> RETURN [order 3] : [deltaI/deltaV == -Iavg/Vavg]
  (junction 16) -> DECREMENT [order 1] : [deltaI/deltaV > -Iavg/Vavg]
  (junction 17) -> DECREMENT [order 2] : [deltaI > 0]
  (junction 16) -> INCREMENT [order 2] : [deltaI/deltaV < -Iavg/Vavg]
  DECREMENT -> RETURN
  INCREMENT -> RETURN
  data: V input; I input; D output double =0.7; k local double; Iavg local double; Iprev local double; Isum local double; Vavg local double; Vprev local double; Vsum local double; d local double; deltaI local double; deltaV local double; deltad local double =8e-3
  events: clk input RISING_EDGE_EVENT

== stateflow chart simscape_final/DC-DC MPPT Boost/P&O Method/P&O Method ==
  state AVERAGE100SAMPLES
    entry:
    P = V*I; Psum = 0; Vsum = 0; k = 0;
    during:
    Psum = Psum +P; Vsum = Vsum + V; k++;
    exit:
    Pavg = Psum/k; Vavg = Vsum/k;
  state SAMPLEandCALCULATE
    entry:
    deltaP = Pavg - Pprev;
    deltaV = Vavg - Vprev;
    d = D;
  state DECREMENT
    entry:
    d = d - deltad;
  state INCREMENT
    entry:
    d = d + deltad;
  state RETURN
    entry:
    Pprev = Pavg; Vprev = Vavg; D = d;
  RETURN -> AVERAGE100SAMPLES
  (default) -> AVERAGE100SAMPLES
  AVERAGE100SAMPLES -> SAMPLEandCALCULATE : after(100,clk)
  SAMPLEandCALCULATE -> RETURN [order 1] : [deltaP==0]
  SAMPLEandCALCULATE -> (junction 138) [order 3] : [deltaP < 0]
  SAMPLEandCALCULATE -> (junction 139) [order 2] : [deltaP >0]
  (junction 139) -> INCREMENT [order 1] : [deltaV < 0]
  (junction 138) -> DECREMENT [order 2] : [deltaV < 0]
  (junction 139) -> DECREMENT [order 2] : [deltaV > 0]
  (junction 138) -> INCREMENT [order 1] : [deltaV > 0]
  DECREMENT -> RETURN
  INCREMENT -> RETURN
  data: V input; I input; D output double =0.7; k local double; Vavg local double; Vprev local double; Vsum local double; d local double; deltaV local double; deltad local double =8e-3; P local double; Pavg local double; Pprev local double; Psum local double; deltaP local double
  events: clk input RISING_EDGE_EVENT

== matlab function simscape_final/MATLAB Function ==
  settings: updateMethod=DISCRETE
  data: Vpv input; D output; Ipv input
%___________________________________________________________________%
%  Grey Wolf Optimizer (GWO) for PV system under PSC                %
%                                                                   %
%  Developed in MATLAB R2021b                                       %
%                                                                   %
%       Detect Vpv and Ipv from the solar panel as input            %
%               to the function                                     %
%                                                                   %
%       Returns Duty cycle as output for the switching device       %
%                in the boost converter                             %
%___________________________________________________________________%
function D = GWO_code(Vpv,Ipv)
persistent u;
persistent d_current;
persistent pbest;
persistent p;
persistent dc;
persistent v;
persistent count;
persistent gbest;
if(isempty(count))
    count=0;
end
if(isempty(d_current))
    d_current=0.9;
end
if(isempty(gbest))
    gbest=0.9;
end
if(isempty(p))
    p=zeros(4,1);
end

if(isempty(v))
    v=zeros(4,1);
end

if(isempty(pbest))
    pbest=zeros(4,1);
end
if(isempty(u))
    u=0;
end
if(isempty(dc))
    dc=zeros(4,1);
    dc(1)=0;
    dc(2)=0.1;
    dc(3)=0.5;
    dc(4)=0.5;
end
if(count>=1 && count<300)
    D=d_current;
    count=count+1;
    return;
end
count=0;

if(u>=1 && u<=4)
    if((Vpv*Ipv)>p(u))
        p(u)=Vpv*Ipv;
        pbest(u)=d_current;
    end
end
u=u+1;
if(u==6)
    u=1;
end
if(u==1)
    D=dc(u);
    d_current=D;
    count=1;
    return;
elseif(u==2)
    D=dc(u);
    d_current=D;
    count=1;
    return;
elseif(u==3)
    D=dc(u);
    d_current=D;
    count=1;
    return;
elseif(u==4)
    D=dc(u);
    d_current=D;
    count=1;
    return;
elseif(u==5 )
    [m,i]=max(p);
    gbest=pbest(i);
    D=gbest;
    d_current=D;
    count=1;
    %update velocity
    v(1)=updatevelocity(pbest(1),dc(1));
    v(2)=updatevelocity(pbest(2),dc(2));
    v(3)=updatevelocity(pbest(3),dc(3));
    v(4)=updatevelocity(pbest(4),dc(4));
    %update duty cycle
    dc(1)=updateduty(v(1),gbest);
    dc(2)=updateduty(v(2),gbest);
    dc(3)=updateduty(v(3),gbest);
    dc(4)=updateduty(v(4),gbest);
    
    return;
    
else
    D=0.1;
    
end


end
function velocity_final = updatevelocity(p_best,d)
r2 = rand;
C = 2*r2;    % C = 2 * r2 where r2 is a random vector with value between 1 and 0
velocity_final = (C*p_best-d);
end
function duty_final = updateduty(velocity,g_best)
r1 = rand;
A = 2*0.1*r1-0.1;   % A = 2 * 0.1 * r1 - 0.1 where r1 is a random vector with value between 1 and 0
d1 = g_best-A*velocity;   % D1 = D(alpha) - A * E where D is the postition vector of a particular grey wolf
if(d1>1)
    duty_final = 1;
elseif(d1<0.1)
    duty_final = 0.1;
else
    duty_final = d1;
end
end
